simulink model "Sim_localization_template"  (R2024b)
settings: Solver=VariableStepAuto  StartTime=0.0  StopTime=T_SIM  MaxStep=0.001  RelTol=1e-3
values from neighbouring files (symbols this model uses):
  d = 0.165    [EX_opt_1.m]    (also in id_LEO.m; init_localization.m; init_localization_template.m; script_init_localization.m)
  D = diag([0.001, 0.001, 0.0175/6, 0.0175/6, 0.0175/6, 0.0175/6*T_s, 0.0175/6*T_s].^2)    [EX_opt_1.m]    (also in init_localization.m; init_localization_template.m; script_init_localization.m)
  d_actual = 0.164    [EX_opt_1.m]    (also in data_for_identification.mat = 0.165; init_localization.m; init_localization_template.m; script_init_localization.m)
  P_INIT_EKF = diag([0.001, 0.001, 0.0175/6, 0.0175/6, 0.0175/6, 0.0175/6*T_s, 0.0175/6*T_s].^2)    [EX_opt_1.m]    (also in init_localization.m; init_localization_template.m; script_init_localization.m)
  PHI_INIT = [0;0]    [EX_opt_1.m]    (also in data_for_identification.mat = [0 0]; id_LEO.m; init_localization.m; init_localization_template.m)
  Q_INIT = q(:,1)    [EX_opt_1.m]    (also in data_for_identification.mat = [0 0 0.463647609001]; id_LEO.m; init_localization.m = [0;0;0]; script_init_localization.m)
  Q_INIT_LOC = Q_INIT    [EX_opt_1.m]    (also in init_localization.m = [0;0;0]; script_init_localization.m = Q_INIT + [0.2; 0.2; deg2rad(15)])
  r = 0.03    [EX_opt_1.m]    (also in id_LEO.m; init_localization.m; init_localization_template.m; script_init_localization.m)
  R_2 = diag([ENCODER_QUANTIZATION/6, ENCODER_QUANTIZATION/6].^2)    [EX_opt_1.m]    (also in init_localization.m = diag([ENCODER_QUANRIZATION/6,ENCODER_QUANRIZATION/6].^2); init_localization_template.m = diag([ENCODER_QUANRIZATION/6,ENCODER_QUANRIZATION/6].^2); script_init_localization.m = diag([ENCODER_QUANRIZATION/6,ENCODER_QUANRIZATION/6].^2))
  R_4 = diag([noise_std, noise_std, ENCODER_QUANTIZATION/6, ENCODER_QUANTIZATION/6].^2)    [EX_opt_1.m]    (also in init_localization.m = diag(([0.001, 0.001, ENCODER_QUANRIZATION/6,ENCODER_QUANRIZA; init_localization_template.m = diag(([0.001, 0.001, ENCODER_QUANRIZATION/6,ENCODER_QUANRIZA; script_init_localization.m = diag(([0.001, 0.001, ENCODER_QUANRIZATION/6,ENCODER_QUANRIZA)
  r_actual = 0.031    [EX_opt_1.m]    (also in data_for_identification.mat = 0.03; init_localization.m; init_localization_template.m; script_init_localization.m)
  T_s = 0.04    [EX_opt_1.m]    (also in EX_opt_2.m = Ts_values(i); data_for_identification.mat; id_LEO.m; id_template.m)
  Z_INIT_EKF = [Q_INIT_LOC; 0; 0; 0; 0]    [EX_opt_1.m]    (also in init_localization.m = [0;0;0])
settings Model: Creator=alberto  LastModifiedBy=alber
settings RTWCC: GPUComputeCapability=3.5

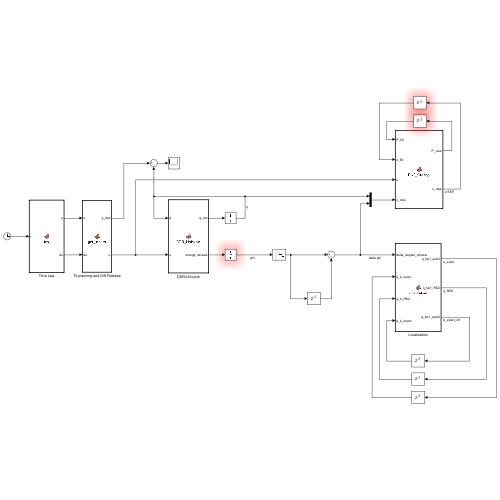
[thumbnail: Simulink's stored preview of the top-level diagram]
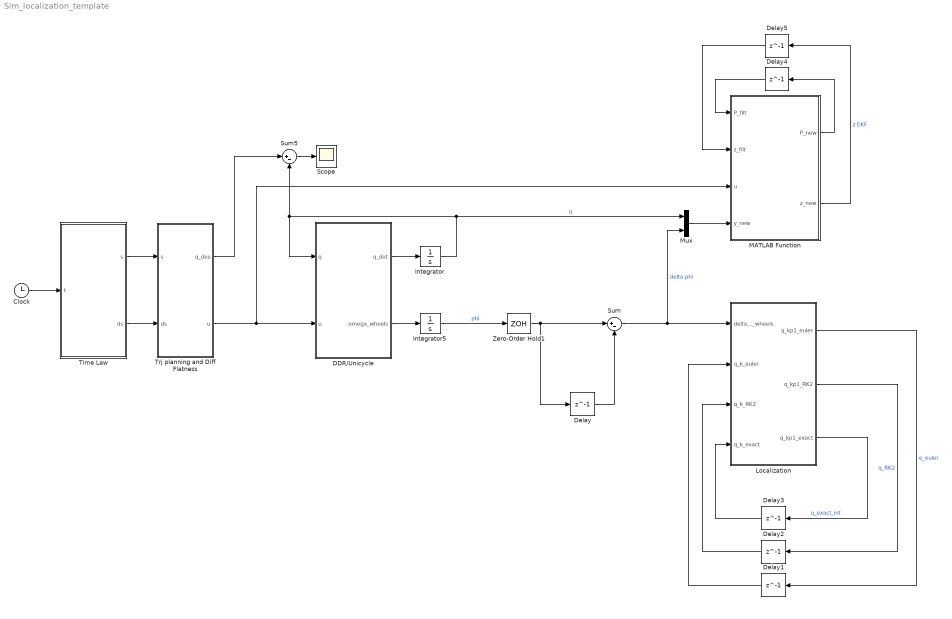
== system Sim_localization_template ==
  Clock : Clock
  DDR/Unicycle : MATLAB Function  TreatAsAtomicUnit=on
  Delay : Delay  DelayLength=1  InitialCondition=[0;0]  SampleTime=T_s
  Delay1 : Delay  DelayLength=1  InitialCondition=Q_INIT_LOC
  Delay2 : Delay  DelayLength=1  InitialCondition=Q_INIT_LOC
  Delay3 : Delay  DelayLength=1  InitialCondition=Q_INIT_LOC
  Delay4 : Delay  DelayLength=1  InitialCondition=P_INIT_EKF  SampleTime=T_s
  Delay5 : Delay  DelayLength=1  InitialCondition=Z_INIT_EKF  SampleTime=T_s
  Integrator : Integrator  InitialCondition=Q_INIT
  Integrator5 : Integrator  InitialCondition=PHI_INIT
  Localization : MATLAB Function  TreatAsAtomicUnit=on
  MATLAB Function : MATLAB Function  TreatAsAtomicUnit=on
  Mux : Mux  Inputs=2
  Scope : Scope
  Sum : Sum  Inputs=|+-
  Sum5 : Sum  Inputs=|+-
  Time Law : MATLAB Function  TreatAsAtomicUnit=on
  Trj planning and Diff Flatness : MATLAB Function  TreatAsAtomicUnit=on
  Zero-Order Hold1 : ZeroOrderHold  SampleTime=T_s
  wires:
  Clock/1 -> Time Law/1(t)
  Trj planning and Diff Flatness/2(u) -> DDR/Unicycle/2(u), MATLAB Function/3(u)
  Zero-Order Hold1/1 -> Sum/1, Delay/1
  Delay/1 -> Sum/2
  Delay1/1 -> Localization/2(q_k_euler)
  Sum/1 -> Mux/2, Localization/1(delta_angles_wheels)  "delta phi"
  Localization/1(q_kp1_euler) -> Delay1/1  "e_euler"
  Integrator/1 -> Mux/1, Sum5/2, DDR/Unicycle/1(q)  "q"
  Delay3/1 -> Localization/4(q_k_exact)
  Delay2/1 -> Localization/3(q_k_RK2)
  Localization/2(q_kp1_RK2) -> Delay2/1  "q_RK2"
  Localization/3(q_kp1_exact) -> Delay3/1  "q_exact_int"
  Time Law/1(s) -> Trj planning and Diff Flatness/1(s)
  Time Law/2(ds) -> Trj planning and Diff Flatness/2(ds)
  DDR/Unicycle/1(q_dot) -> Integrator/1
  Trj planning and Diff Flatness/1(q_des) -> Sum5/1
  Sum5/1 -> Scope/1
  DDR/Unicycle/2(omega_wheels) -> Integrator5/1
  Integrator5/1 -> Zero-Order Hold1/1  "phi"
  MATLAB Function/1(P_new) -> Delay4/1
  Delay4/1 -> MATLAB Function/1(P_filt)
  Delay5/1 -> MATLAB Function/2(z_filt)
  MATLAB Function/2(z_new) -> Delay5/1  "z EKF"
  Mux/1 -> MATLAB Function/4(y_new)

== matlab function Sim_localization_template/Time Law ==
  data: t input; s output; ds output
function [s, ds] = fcn(t)

== matlab function Sim_localization_template/DDR//Unicycle ==
  data: q input; u input; q_dot output; omega_wheels output; d_actual parameter; r_actual parameter
function [q_dot, omega_wheels] = DDR_Unicycle(q, u, d_actual, r_actual)

== matlab function Sim_localization_template/Trj planning and Diff Flatness ==
  data: q_des output; s input; u output; ds input
function [q_des, u] = get_inputs(s, ds)

== matlab function Sim_localization_template/Localization ==
  data: delta_angles_wheels input; q_k_euler input; q_k_RK2 input; q_k_exact input; r parameter; d parameter; q_kp1_euler output; T_s parameter; q_kp1_RK2 output; q_kp1_exact output
function [q_kp1_euler, q_kp1_RK2, q_kp1_exact] = localization(delta_angles_wheels, q_k_euler, q_k_RK2, q_k_exact, r, d, T_s)

== matlab function Sim_localization_template/MATLAB Function ==
  data: P_filt input; P_new output; z_filt input; z_new output; u input; y_new input; D parameter; R_2 parameter; R_4 parameter; T_s parameter; r parameter; d parameter
function [P_new, z_new] = EKF_filtering(P_filt, z_filt, u, y_new, D, R_2, R_4, T_s, r, d)
